simulink model "model"  (R2021a)
settings: Solver=ode15s  StartTime=0.0  StopTime=120  RelTol=1e-3
values from neighbouring files (symbols this model uses):
  Bf = 0.0001    [params.mat]
  CQ0 = 3.10795972642e-07    [params.mat]
  CQ1 = -4.88223811566e-06    [params.mat]
  CT0 = 5.09126113853e-06    [params.mat]
  CT1 = -6.35871877158e-05    [params.mat]
  Jt = 2.71171110304e-06    [params.mat]
  Ke = 0.000179294405789    [params.mat]
  La = 0.0600029561553    [params.mat]
  Ra = 1    [params.mat]
  Td = 0.04318    [params.mat]
settings Model: Creator=gpob  LastModifiedBy=gpob

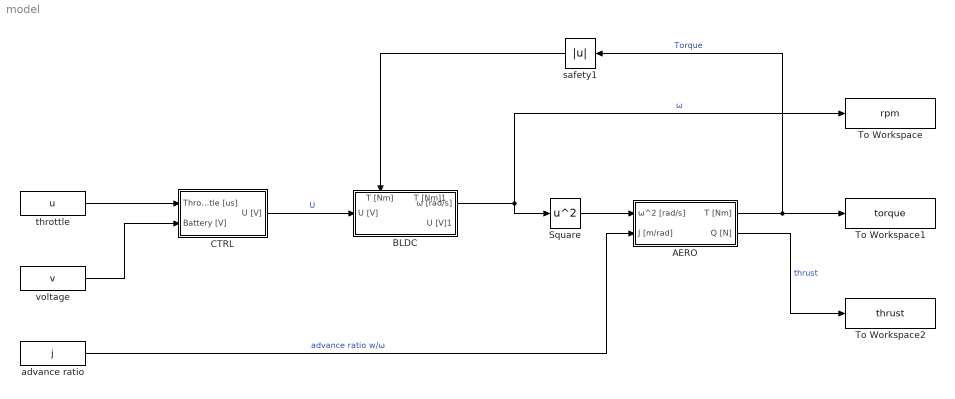
== system model ==
  AERO : Subsystem
  BLDC : Subsystem
      settings: PortSchema="{\"entries\":[{\"content\":{\"sides\":[{\"content\":{\"connectorIds\":[\"In1\"]},\"type\":\"ConnectorPlacement.EquallySpacedRectSide\",\"uuid\":\"274ecf24-0b1f-4e48-9e8c-283c14986efc\"},{\"content\":{\"connectorIds\":[\"Out1\",\"Out2\"],\"side\":\"RIGHT\"},\"type\":\"ConnectorPlacement.EquallySpacedRectSide\",\"uuid\":\"d2296534-28d8-4f9c-a8d5-908cd34053db\"},{\"content\":{\"connectorIds\":[\"In2\",\"In3\"],\"side\":\"TOP\"},\"type\":\"ConnectorPlacement.EquallySpacedRectSide\",\"uuid\":\"0642ca32-8524-4238-bc0e-89fea8dfc158\"}]},\"type\":\"ConnectorPlacement.EquallySpacedConnector\",\"uuid\":\"4dc4e53c-7bd2-4fbc-a3d3-c126dfc0eebc\"}],\"packageUris\":[\"http://schema.mathworks.com/mf0/Connector/R2020b\"],\"version\":\"1.0\"}"
  CTRL : Subsystem
  Square : Math  Operator=square  SaturateOnIntegerOverflow=on
  To Workspace : ToWorkspace  VariableName=rpm  SaveFormat=Timeseries  SampleTime=-1
  To Workspace1 : ToWorkspace  VariableName=torque  SaveFormat=Timeseries  SampleTime=-1
  To Workspace2 : ToWorkspace  VariableName=thrust  SaveFormat=Timeseries  SampleTime=-1
  advance ratio : FromWorkspace  VariableName=j
  safety1 : Abs
  throttle : FromWorkspace  VariableName=u
  voltage : FromWorkspace  VariableName=v
  wires:
  throttle/1 -> CTRL/1(Throttle [us])
  Square/1 -> AERO/1(ω^2 [rad/s])
  voltage/1 -> CTRL/2(Battery [V])
  AERO/1(T [Nm]) -> safety1/1, To Workspace1/1  "Torque"
  advance ratio/1 -> AERO/2(J [m/rad])  "advance ratio w/ω"
  AERO/2(Q [N]) -> To Workspace2/1  "thrust"
  safety1/1 -> BLDC/2(T [Nm])
  BLDC/1(ω [rad/s]) -> Square/1, To Workspace/1  "ω"
  CTRL/1(U [V]) -> BLDC/1(U [V])  "U"

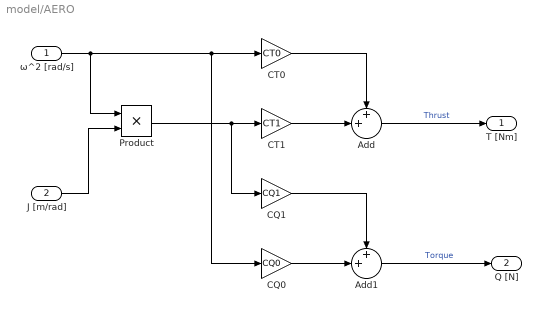
== system model/AERO ==
  ω^2 [rad/s] : Inport
  J [m/rad] : Inport  Port=2
  Add : Sum  Inputs=++|
  Add1 : Sum  Inputs=++|
  CQ0 : Gain  Gain=CQ0
  CQ1 : Gain  Gain=CQ1
  CT0 : Gain  Gain=CT0
  CT1 : Gain  Gain=CT1
  Product : Product
  T [Nm] : Outport
  Q [N] : Outport  Port=2
  wires:
  J [m/rad]/1 -> Product/2
  Product/1 -> CQ1/1, CT1/1
  ω^2 [rad/s]/1 -> Product/1, CQ0/1, CT0/1
  CT1/1 -> Add/2
  Add/1 -> T [Nm]/1  "Thrust"
  CT0/1 -> Add/1
  Add1/1 -> Q [N]/1  "Torque"
  CQ1/1 -> Add1/1
  CQ0/1 -> Add1/2

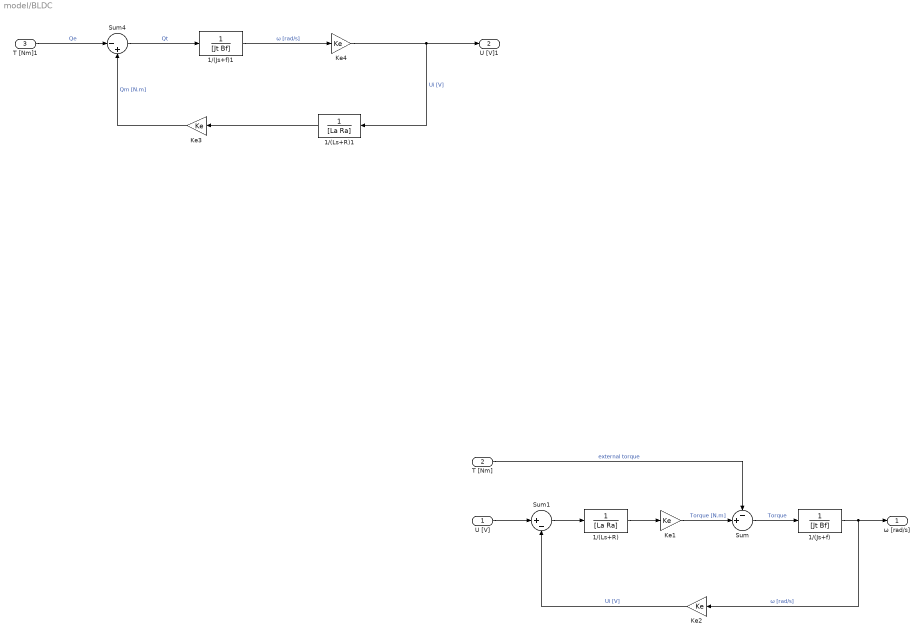
== system model/BLDC ==
  U [V] : Inport
  T [Nm] : Inport  Port=2
  T [Nm]1 : Inport  Port=3
  1/(Js+f) : TransferFcn  Denominator=[Jt Bf]
  1/(Js+f)1 : TransferFcn  Denominator=[Jt Bf]
  1/(Ls+R) : TransferFcn  Denominator=[La Ra]
  1/(Ls+R)1 : TransferFcn  Denominator=[La Ra]
  Ke{1..4} (4 alike) : Gain  Gain=Ke
  Sum : Sum  Inputs=-+|
  Sum1 : Sum  Inputs=|+-
  Sum4 : Sum  Inputs=|-+
  ω [rad/s] : Outport
  U [V]1 : Outport  Port=2
  wires:
  Sum/1 -> 1/(Js+f)/1  "Torque"
  T [Nm]/1 -> Sum/1  "external torque"
  1/(Js+f)/1 -> Ke2/1, ω [rad/s]/1  "ω [rad/s]"
  Sum1/1 -> 1/(Ls+R)/1
  U [V]/1 -> Sum1/1
  Ke2/1 -> Sum1/2  "Ui [V]"
  1/(Ls+R)/1 -> Ke1/1
  Ke1/1 -> Sum/2  "Torque [N.m]"
  Ke3/1 -> Sum4/2  "Qm [N.m]"
  1/(Ls+R)1/1 -> Ke3/1
  1/(Js+f)1/1 -> Ke4/1  "ω [rad/s]"
  T [Nm]1/1 -> Sum4/1  "Qe"
  Sum4/1 -> 1/(Js+f)1/1  "Qt"
  Ke4/1 -> U [V]1/1, 1/(Ls+R)1/1  "Ui [V]"

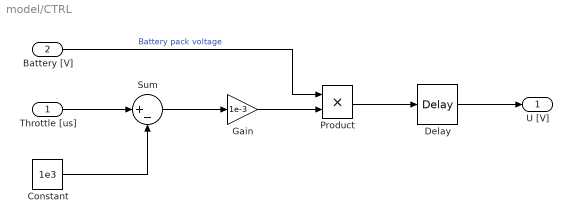
== system model/CTRL ==
  Throttle [us] : Inport
  Battery [V] : Inport  Port=2
  Constant : Constant  Value=1e3
  Delay : TransportDelay  DelayTime=Td
  Gain : Gain  Gain=1e-3
  Product : Product  Inputs=**
  Sum : Sum  Inputs=|+-
  U [V] : Outport
  wires:
  Battery [V]/1 -> Product/1  "Battery pack voltage"
  Constant/1 -> Sum/2
  Sum/1 -> Gain/1
  Gain/1 -> Product/2
  Throttle [us]/1 -> Sum/1
  Product/1 -> Delay/1
  Delay/1 -> U [V]/1
